simulink subsystem "EKF"  (R2024a)
settings: Solver=VariableStepAuto  StartTime=0.0  StopTime=10.0  RelTol=1e-3
undefined symbols (not defined in the file): N_KF, Q_KF, R_KF, x_eq
settings Model: Creator=Bocchio  LastModifiedBy=Bocchio

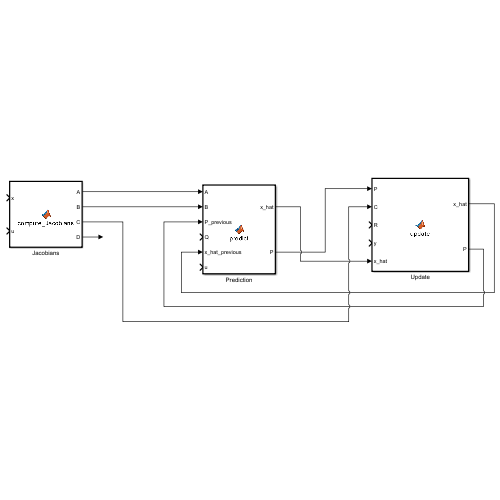
[thumbnail: Simulink's stored preview of the top-level diagram]
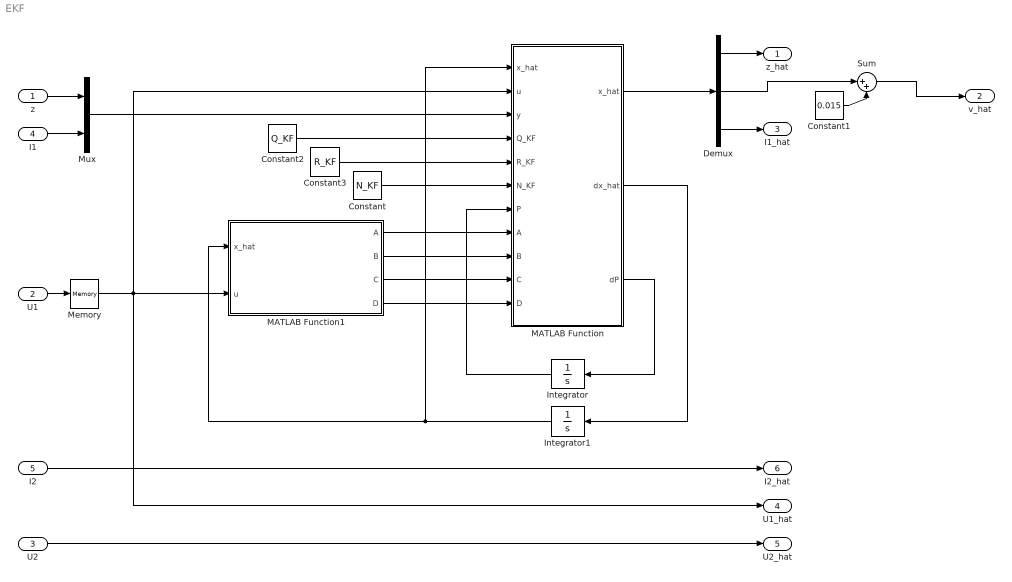
== system EKF ==
  z : Inport
  U1 : Inport  Port=2
  U2 : Inport  Port=3
  I1 : Inport  Port=4
  I2 : Inport  Port=5
  Constant : Constant  Value=N_KF
  Constant1 : Constant  Value=0.015
  Constant2 : Constant  Value=Q_KF
  Constant3 : Constant  Value=R_KF
  Demux : Demux  Outputs=3
  Integrator : Integrator  InitialCondition=zeros(3, 3)
  Integrator1 : Integrator  InitialCondition=x_eq
  MATLAB Function : MATLAB Function  TreatAsAtomicUnit=on
  MATLAB Function1 : MATLAB Function  TreatAsAtomicUnit=on
  Memory : Memory
  Mux : Mux  Inputs=2
  Sum : Sum  Inputs=|++
  z_hat : Outport
  v_hat : Outport  Port=2
  I1_hat : Outport  Port=3
  U1_hat : Outport  Port=4
  U2_hat : Outport  Port=5
  I2_hat : Outport  Port=6
  wires:
  MATLAB Function1/3(C) -> MATLAB Function/10(C)
  U1/1 -> Memory/1
  MATLAB Function1/2(B) -> MATLAB Function/9(B)
  Constant2/1 -> MATLAB Function/4(Q_KF)
  MATLAB Function1/1(A) -> MATLAB Function/8(A)
  MATLAB Function/2(dx_hat) -> Integrator1/1
  U2/1 -> U2_hat/1
  Demux/3 -> I1_hat/1
  z/1 -> Mux/1
  I1/1 -> Mux/2
  Mux/1 -> MATLAB Function/3(y)
  MATLAB Function1/4(D) -> MATLAB Function/11(D)
  Constant3/1 -> MATLAB Function/5(R_KF)
  Constant/1 -> MATLAB Function/6(N_KF)
  MATLAB Function/1(x_hat) -> Demux/1
  I2/1 -> I2_hat/1
  MATLAB Function/3(dP) -> Integrator/1
  Integrator/1 -> MATLAB Function/7(P)
  Integrator1/1 -> MATLAB Function1/1(x_hat), MATLAB Function/1("x_hat ")
  Memory/1 -> MATLAB Function/2(u), MATLAB Function1/2(u), U1_hat/1
  Demux/2 -> Sum/1
  Constant1/1 -> Sum/2
  Demux/1 -> z_hat/1
  Sum/1 -> v_hat/1

== matlab function EKF/MATLAB Function ==
  data: x_hat output; x_hat input; u input; dx_hat output; y input; dP output; Q_KF input; R_KF input; N_KF input; P input; A input; B input; C input; D input
function [x_hat, dx_hat, dP]  = EKF(x_hat, u, y, Q_KF, R_KF, N_KF, P, A, B, C, D)

G = [0 0; 1 0; 0 1];
H = zeros(2, 2);

% Computing R_bar and N_bar
R_bar = R_KF + H*N_KF + N_KF'*H' + H*Q_KF*H';
N_bar = G * (Q_KF*H' + N_KF);


%% Prediction and  update

% ARE
P = reshape(P, size(A));
dP = (A*P + P*A' + [B G]*blkdiag(0, Q_KF)*[B G]' - P*C'* R_KF^-1 *C*P);

% Optimal gain
K = (P*C' + N_bar) / R_bar;

dx_hat = A*x_hat + B*u + K*(y - C*x_hat);

end

== matlab function EKF/MATLAB Function1 ==
  settings: updateMethod=DISCRETE
  data: A output; B output; C output; D output; x_hat input; u input
function [A, B, C, D] = ABCD_lagrangian_1DOF(x_hat, u)

%% Parameters

% Physical constants
g = 9.81; %[m/s^2]
m = 60.54 * 1e-3; %[kg]

% Current model
V1min = 4.300000e-02; %[V]
k1 = +1.165800e+01; %[V/MU]
c1 = -5.608000e-01; %[V]
PWM_min = 5.179276/100; %[MU]

% Inductances
L10 = 6.539244e-02; %[H]
a1z = 1.585423e+02; %[1/m]
L1z = 4.044743e-02; %[H]
a1I = 5.296552e+00; %[]
b1I = 1.042271e+00; %[A]
L1I = 3.288792e-02; %[H]

% Resistances
R10 = 4.17; %[ohm]


%% ABCD for Kalman filter computation

voltage = @(PWM) ...
    (PWM < PWM_min) .* (V1min) + ...
    (PWM >= PWM_min) .* (k1 * PWM + c1);

L1 = @(x, I) L10 + L1z * exp(-a1z*x) + L1I * atan(a1I * I - b1I);
dL1dx = @(x) -a1z*L1z * exp(-a1z*x);
dL1ddx = @(x) +a1z^2*L1z * exp(-a1z*x);

% A coefficients
a11 = 0;
a12 = 1;
a13 = 0;

a21 = 1 / m * (1/2 * dL1ddx(x_hat(1)) * x_hat(3)^2);
a22 = 0;
a23 = 1 / m * dL1dx(x_hat(1)) * x_hat(3);

a31 = -1 / L1(x_hat(1), x_hat(3))^2 * dL1dx(x_hat(1)) * (-R10 * x_hat(3) + voltage(u(1)));
a32 = 0;
a33 = 1 / L1(x_hat(1), x_hat(3)) * (-R10);

% B coefficients
b11 = 0;
b21 = 0;
b31 = 1 / L1(x_hat(1), x_hat(3)) * k1;

% C coefficients
c1 = 1;
c2 = 0;
c3 = 0;

% D coefficients
d1 = 0;


% State matrices
A = [
    a11 a12 a13;
    a21 a22 a23;
    a31 a32 a33
    ];

B = [
    b11
    b21
    b31
    ];

C = [
    1 0 0;
    0 0 1
    ];

D = d1;

end
